simulink model "PMSMqidong_succeed"  (R2016a)
settings: Solver=ode15s  StartTime=0.0  StopTime=1  MaxStep=1e-5  RelTol=1e-3
libraries: powerlib x5
settings Model: Creator=84360  LastModifiedBy=user

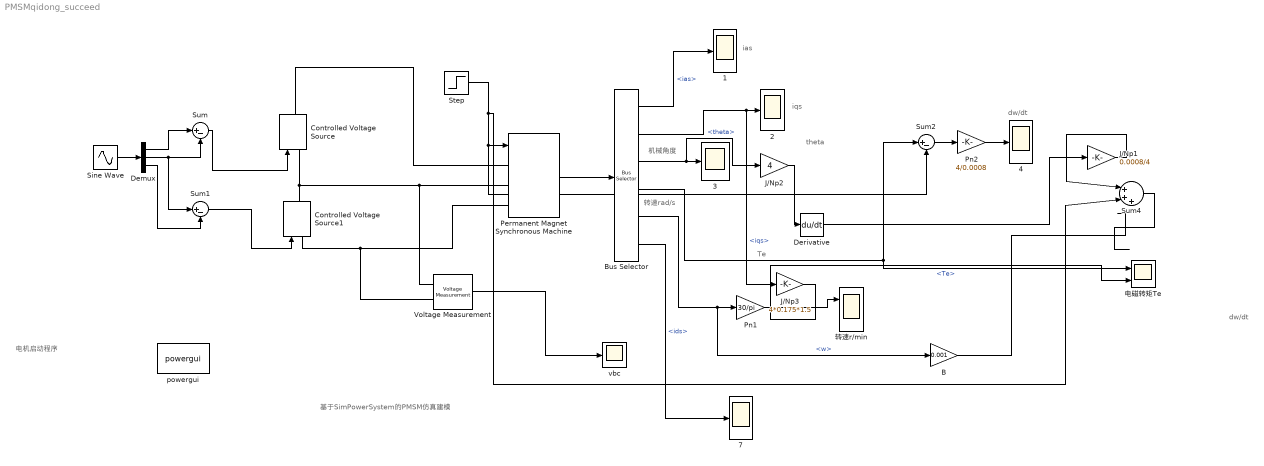
== system PMSMqidong_succeed ==
  note: dw/dt
  note: dw/dt
  note: 机械角度
  note: 转速rad/s
  note: 基于SimPowerSystem的PMSM仿真建模
  note: theta
  note: iqs
  note: ias
  note: Te
  note: 电机启动程序
  {1..4,7} (5 alike) : Scope
  B : Gain  Gain=0.001
  Bus Selector : BusSelector  OutputSignals=ias,iqs,theta,Te,w,ids
  Controlled Voltage Source : powerlib/Electrical Sources/Controlled Voltage Source  Initialize=on  Source_Type=AC  Amplitude=0  Phase=0  Frequency=0  Measurements=None
  Controlled Voltage Source1 : powerlib/Electrical Sources/Controlled Voltage Source  Initialize=on  Source_Type=AC  Amplitude=0  Phase=0  Frequency=0  Measurements=None
  Demux : Demux  Outputs=3
  Derivative : Derivative
  J/Np1 : Gain  Gain=0.0008/4
  J/Np2 : Gain  Gain=4
  J/Np3 : Gain  Gain=4*0.175*1.5
  Permanent Magnet Synchronous Machine : powerlib/Machines/Permanent Magnet Synchronous Machine  NbPhases=3  FluxDistribution=Sinusoidal  RotorType=Salient-pole  MechanicalLoad=Torque Tm  PresetModel=No  ShowDetailedParameters=on  MeasurementBus=on  Resistance=2.8750  Inductance=8.5e-3  dqInductances=[8.5e-3,8.5e-3]  La=0.000395  MachineConstant=Flux linkage established by magnets (V.s)  Flux=0.175  VoltageCst=126.966  TorqueCst=1.05  Flat=120  Mechanical=[0.0008 0.001 4 0]  PolePairs=4  InitialConditions=[0,0, 0,0]  InitialConditions5ph=[0 0 0 0 0 0]  TsPowergui=0  TsBlock=-1  RefAngle=Aligned with phase A axis (original Park)
  Pn1 : Gain  Gain=30/pi
  Pn2 : Gain  Gain=4/0.0008
  Sine Wave : Sin  Amplitude=220*sqrt(2)  Frequency=80*pi  Phase=[0 -2*pi/3 2*pi/3]-[-pi/2 -pi/2 -pi/2]  SampleTime=0
  Step : Step  Time=0.3  Before=1  After=5  SampleTime=0
  Sum : Sum  Inputs=|+-
  Sum1 : Sum  Inputs=|+-
  Sum2 : Sum  Inputs=|+-
  Sum4 : Sum  Inputs=|+++
  Voltage Measurement : powerlib/Measurements/Voltage Measurement  PhasorSimulation=off  OutputType=Complex  PSBequivalent=0
  powergui : powerlib/powergui  Priority=1  SimulationMode=Continuous  SolverType=Tustin/Backward Euler (TBE)  SampleTime=50e-6  frequency=60  SPID=off  DisableSnubberDevices=off  DisableRonSwitches=off  DisableVfSwitches=off  SwTol=0  DisplayEquations=off  Interpol=off  ExternalGateDelay=off  methode=off  Ts=10  FunctionMessages=off  echomessages=off  HookPort=off  EnableUseOfTLC=off  x0status=blocks  frequencyindice=0  Pbase=100e6  ErrMax=1e-4  Iterations=50  UnitsV=kV  UnitsW=MW  buscounter=0  RestoreLinks=warning  ResistiveCurrentMeasurement=off  Frange=[0:2:500]  Ylog=off  Xlog=on  ShowGrid=off  save=off  variable=ZData  structure=0  ZoomFFT=off  StartTime=0.0  cycles=1  DisplayStyle=1  fundamental=60  FreqAxis=off  MaxFrequency=1000  frequencyindicesteady=1  RmsSteady=1  display=off
  vbc : Scope
  电磁转矩Te : Scope  NumInputPorts=2
  转速r/min : Scope  NumInputPorts=2
  wires:
  Permanent Magnet Synchronous Machine/1 -> Bus Selector/1
  Step/1 -> Sum4/2, Sum2/2, Permanent Magnet Synchronous Machine/1
  Sum/1 -> Controlled Voltage Source/1
  Sum1/1 -> Controlled Voltage Source1/1
  Voltage Measurement/1 -> vbc/1
  Bus Selector/1 -> 1/1  "<ias>"
  Bus Selector/2 -> J/Np3/1, 2/1  "<iqs>"
  Bus Selector/3 -> J/Np2/1, 3/1  "<theta>"
  Bus Selector/4 -> Sum2/1, 电磁转矩Te/1  "<Te>"
  Bus Selector/5 -> B/1, Pn1/1  "<w>"
  Bus Selector/6 -> 7/1  "<ids>"
  Sine Wave/1 -> Demux/1
  Demux/1 -> Sum/1
  Demux/2 -> Sum/2, Sum1/1
  Demux/3 -> Sum1/2
  Pn1/1 -> 转速r/min/1
  Sum2/1 -> Pn2/1
  Pn2/1 -> 4/1
  B/1 -> ?
  Sum4/1 -> ?
  J/Np1/1 -> Sum4/1
  J/Np2/1 -> Derivative/1
  Derivative/1 -> J/Np1/1
  J/Np3/1 -> 电磁转矩Te/2
  connections:
  Controlled Voltage Source1/RConn1 -- Controlled Voltage Source/LConn1 -- Voltage Measurement/LConn1 -- Permanent Magnet Synchronous Machine/LConn2
  Controlled Voltage Source/RConn1 -- Permanent Magnet Synchronous Machine/LConn1
  Controlled Voltage Source1/LConn1 -- Voltage Measurement/LConn2 -- Permanent Magnet Synchronous Machine/LConn3
